simulink model "SmithPredictorEinstellen"  (R2018b)
settings: Solver=VariableStepAuto  StartTime=0.0  StopTime=900*10  FixedStep=0.1  RelTol=1e-3
undefined symbols (not defined in the file or in its folder): s
libraries: cstblocks x12, simulink x6
settings Model: Creator=Adrian Gehrig  LastModifiedBy=Trips
settings SFSimCC: SimUseLocalCustomCode=off
settings RTWCC: RTWUseLocalCustomCode=off
settings CodeAppCC: StateflowObjectComments=on

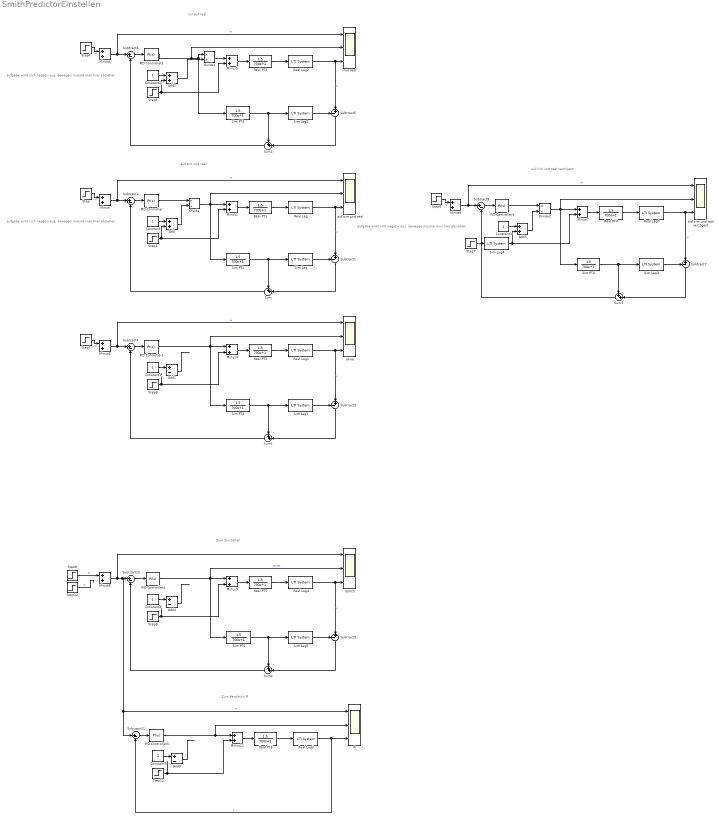
== system SmithPredictorEinstellen ==
  note: Zum Einstellen
  note: nur auf real
  note: aufgabe wirkt sich negativ aus, dewegen müsste man hier abziehen
  note: aufgabe wirkt sich negativ aus, dewegen müsste man hier abziehen
  note: auf sim und real
  note: aufgabe wirkt sich negativ aus, dewegen müsste man hier abziehen
  note: auf sim und real verzögert
  note: Zum Vergleich PI
  Add : Sum
  Add1 : Sum  Inputs=+-
  Add2 : Sum
  Add3 : Sum
  Add4 : Sum  Inputs=+-
  Add5 : Sum  Inputs=+-
  Constant{,1..5} (6 alike) : Constant
  Divide : Product  Inputs=*/
  Divide1 : Product  Inputs=*/
  Divide2 : Product  Inputs=*/
  Minus{,1..9,11} (11 alike) : Sum
  PI : Scope  NumInputPorts=3
  PID Controller{,1..3} (4 alike) : simulink/Continuous/PID Controller  Controller=PI  Form=Ideal  TimeDomain=Continuous-time  SampleTime=-1  IntegratorMethod=Forward Euler  FilterMethod=Forward Euler  ControllerParametersSource=internal  P=1  I=0.00482346678976217  D=0  UseFilter=on  N=100  TunerSelectOption=Transfer Function Based (PID Tuner App)  InitialConditionSource=internal  InitialConditionForIntegrator=0  InitialConditionForFilter=0  DifferentiatorICPrevScaledInput=0  ExternalReset=none  TrackingMode=off  Kt=1  LimitOutput=off  UpperSaturationLimit=inf  LowerSaturationLimit=-inf  LinearizeAsGain=on  AntiWindupMode=none  Kb=1  POutMin=[]  POutMax=[]  IOutMin=[]  IOutMax=[]  DOutMin=[]  DOutMax=[]  NOutMin=[]  NOutMax=[]  SumOutMin=[]  SumOutMax=[]  SaturationOutMin=[]  SaturationOutMax=[]  PParamMin=[]  PParamMax=[]  IParamMin=[]  IParamMax=[]  DParamMin=[]  DParamMax=[]  NParamMin=[]  NParamMax=[]  KbParamMin=[]  KbParamMax=[]  KtParamMin=[]  KtParamMax=[]  KbOutMin=[]  KbOutMax=[]  KtOutMin=[]  KtOutMax=[]  IntegratorOutMin=[]  IntegratorOutMax=[]  FilterOutMin=[]  FilterOutMax=[]  SumI1OutMin=[]  SumI1OutMax=[]  SumI2OutMin=[]  SumI2OutMax=[]  SumI3OutMin=[]  SumI3OutMax=[]  SumI4OutMin=[]  SumI4OutMax=[]  SumDOutMin=[]  SumDOutMax=[]  DifferentiatorOutMin=[]  DifferentiatorOutMax=[]  FilterDiffOutCoefMin=[]  FilterDiffOutCoefMax=[]  ReciprocalOutMin=[]  ReciprocalOutMax=[]  SumDenOutMin=[]  SumDenOutMax=[]  SumNumOutMin=[]  SumNumOutMax=[]  DivideOutMin=[]  DivideOutMax=[]  IntegratorContinuousStateAttributes=''  IntegratorStateMustResolveToSignalObject=off  IntegratorRTWStateStorageClass=Auto  FilterContinuousStateAttributes=''  FilterStateMustResolveToSignalObject=off  FilterRTWStateStorageClass=Auto  ParallelPVariant=Passthrough  IdealPVariant=InternalParameters  IVariant=InternalParameters  DVariant=Disabled  IntegratorVariant=Continuous  SatVariant=Disabled  AWVariant=Passthrough  PCopyVariant=Disabled  TRVariant=Disabled  FdbkBlocksVariant=Forward  IdealPFdbkVariant=Disabled  SatFdbkVariant=Disabled  DerivativeFilterVariant=Disabled  NVariant=Disabled  NCopyVariant=Disabled_SignalSpec  FilterICVariant=Disabled  IntegratorICVariant=InternalICs  ExternalResetVariant=Disabled  TRSumVariant=Passthrough  SumFdbkVariant=Disabled  SumVariant=Sum_PI
  PID Controller4 : simulink/Continuous/PID Controller  Controller=PI  Form=Ideal  TimeDomain=Continuous-time  SampleTime=-1  IntegratorMethod=Forward Euler  FilterMethod=Forward Euler  ControllerParametersSource=internal  P=0.3  I=0.00122023353289823  D=0  UseFilter=on  N=100  TunerSelectOption=Transfer Function Based (PID Tuner App)  InitialConditionSource=internal  InitialConditionForIntegrator=0  InitialConditionForFilter=0  DifferentiatorICPrevScaledInput=0  ExternalReset=none  TrackingMode=off  Kt=1  LimitOutput=off  UpperSaturationLimit=inf  LowerSaturationLimit=-inf  LinearizeAsGain=on  AntiWindupMode=none  Kb=1  POutMin=[]  POutMax=[]  IOutMin=[]  IOutMax=[]  DOutMin=[]  DOutMax=[]  NOutMin=[]  NOutMax=[]  SumOutMin=[]  SumOutMax=[]  SaturationOutMin=[]  SaturationOutMax=[]  PParamMin=[]  PParamMax=[]  IParamMin=[]  IParamMax=[]  DParamMin=[]  DParamMax=[]  NParamMin=[]  NParamMax=[]  KbParamMin=[]  KbParamMax=[]  KtParamMin=[]  KtParamMax=[]  KbOutMin=[]  KbOutMax=[]  KtOutMin=[]  KtOutMax=[]  IntegratorOutMin=[]  IntegratorOutMax=[]  FilterOutMin=[]  FilterOutMax=[]  SumI1OutMin=[]  SumI1OutMax=[]  SumI2OutMin=[]  SumI2OutMax=[]  SumI3OutMin=[]  SumI3OutMax=[]  SumI4OutMin=[]  SumI4OutMax=[]  SumDOutMin=[]  SumDOutMax=[]  DifferentiatorOutMin=[]  DifferentiatorOutMax=[]  FilterDiffOutCoefMin=[]  FilterDiffOutCoefMax=[]  ReciprocalOutMin=[]  ReciprocalOutMax=[]  SumDenOutMin=[]  SumDenOutMax=[]  SumNumOutMin=[]  SumNumOutMax=[]  DivideOutMin=[]  DivideOutMax=[]  IntegratorContinuousStateAttributes=''  IntegratorStateMustResolveToSignalObject=off  IntegratorRTWStateStorageClass=Auto  FilterContinuousStateAttributes=''  FilterStateMustResolveToSignalObject=off  FilterRTWStateStorageClass=Auto  ParallelPVariant=Passthrough  IdealPVariant=InternalParameters  IVariant=InternalParameters  DVariant=Disabled  IntegratorVariant=Continuous  SatVariant=Disabled  AWVariant=Passthrough  PCopyVariant=Disabled  TRVariant=Disabled  FdbkBlocksVariant=Forward  IdealPFdbkVariant=Disabled  SatFdbkVariant=Disabled  DerivativeFilterVariant=Disabled  NVariant=Disabled  NCopyVariant=Disabled_SignalSpec  FilterICVariant=Disabled  IntegratorICVariant=InternalICs  ExternalResetVariant=Disabled  TRSumVariant=Passthrough  SumFdbkVariant=Disabled  SumVariant=Sum_PI
  PID Controller5 : simulink/Continuous/PID Controller  Controller=PI  Form=Ideal  TimeDomain=Continuous-time  SampleTime=-1  IntegratorMethod=Forward Euler  FilterMethod=Forward Euler  ControllerParametersSource=internal  P=0.3  I=0.00122496125356266  D=0  UseFilter=on  N=100  TunerSelectOption=Transfer Function Based (PID Tuner App)  InitialConditionSource=internal  InitialConditionForIntegrator=0  InitialConditionForFilter=0  DifferentiatorICPrevScaledInput=0  ExternalReset=none  TrackingMode=off  Kt=1  LimitOutput=off  UpperSaturationLimit=inf  LowerSaturationLimit=-inf  LinearizeAsGain=on  AntiWindupMode=none  Kb=1  POutMin=[]  POutMax=[]  IOutMin=[]  IOutMax=[]  DOutMin=[]  DOutMax=[]  NOutMin=[]  NOutMax=[]  SumOutMin=[]  SumOutMax=[]  SaturationOutMin=[]  SaturationOutMax=[]  PParamMin=[]  PParamMax=[]  IParamMin=[]  IParamMax=[]  DParamMin=[]  DParamMax=[]  NParamMin=[]  NParamMax=[]  KbParamMin=[]  KbParamMax=[]  KtParamMin=[]  KtParamMax=[]  KbOutMin=[]  KbOutMax=[]  KtOutMin=[]  KtOutMax=[]  IntegratorOutMin=[]  IntegratorOutMax=[]  FilterOutMin=[]  FilterOutMax=[]  SumI1OutMin=[]  SumI1OutMax=[]  SumI2OutMin=[]  SumI2OutMax=[]  SumI3OutMin=[]  SumI3OutMax=[]  SumI4OutMin=[]  SumI4OutMax=[]  SumDOutMin=[]  SumDOutMax=[]  DifferentiatorOutMin=[]  DifferentiatorOutMax=[]  FilterDiffOutCoefMin=[]  FilterDiffOutCoefMax=[]  ReciprocalOutMin=[]  ReciprocalOutMax=[]  SumDenOutMin=[]  SumDenOutMax=[]  SumNumOutMin=[]  SumNumOutMax=[]  DivideOutMin=[]  DivideOutMax=[]  IntegratorContinuousStateAttributes=''  IntegratorStateMustResolveToSignalObject=off  IntegratorRTWStateStorageClass=Auto  FilterContinuousStateAttributes=''  FilterStateMustResolveToSignalObject=off  FilterRTWStateStorageClass=Auto  ParallelPVariant=Passthrough  IdealPVariant=InternalParameters  IVariant=InternalParameters  DVariant=Disabled  IntegratorVariant=Continuous  SatVariant=Disabled  AWVariant=Passthrough  PCopyVariant=Disabled  TRVariant=Disabled  FdbkBlocksVariant=Forward  IdealPFdbkVariant=Disabled  SatFdbkVariant=Disabled  DerivativeFilterVariant=Disabled  NVariant=Disabled  NCopyVariant=Disabled_SignalSpec  FilterICVariant=Disabled  IntegratorICVariant=InternalICs  ExternalResetVariant=Disabled  TRSumVariant=Passthrough  SumFdbkVariant=Disabled  SumVariant=Sum_PI
  Real Lag{,1..5} (6 alike) : cstblocks/LTI System  sys=exp(-420*s)  IC=[]
  Real PT{1..6} (6 alike) : TransferFcn  Numerator=[1.5]  Denominator=[700 1]
  Sim Lag{,1..4} (5 alike) : cstblocks/LTI System  sys=exp(-400*s)  IC=[]
  Sim Lag5 : cstblocks/LTI System  sys=exp(-420*s)  IC=[]
  Sim PT{1..5} (5 alike) : TransferFcn  Numerator=[1.5]  Denominator=[700 1]
  Smith : Scope  NumInputPorts=3
  Step{,2,4,6,8} (5 alike) : Step  SampleTime=0
  Step{1,3,5,7,9,11} (6 alike) : Step  Time=5000  SampleTime=0
  Step12 : Step  Time=3000  SampleTime=0
  Subtract{1,3,5,7,9} (5 alike) : Sum  Inputs=-+|
  Subtract{2,4,6,8,10..11} (6 alike) : Sum  Inputs=|+-
  Sum{,1..4} (5 alike) : Sum  Inputs=++|
  "auf sim und real " : Scope  NumInputPorts=3
  auf sim und real verzögert : Scope  NumInputPorts=3
  nur real : Scope  NumInputPorts=3
  ohne : Scope  NumInputPorts=3
  wires:
  Sim PT1/1 -> Sum/1, Sim Lag/1
  Subtract1/1 -> Sum/2
  Sim Lag/1 -> Subtract1/1
  Sum/1 -> Subtract2/2
  Divide/1 -> "auf sim und real "/2, Minus1/1, Sim PT1/1
  Minus/1 -> "auf sim und real "/1, Subtract2/1  "w"
  Subtract2/1 -> PID Controller/1
  Real Lag/1 -> "auf sim und real "/3, Subtract1/2  "y"
  Step/1 -> Minus/1  "w"
  Step1/1 -> Add/2, Minus1/2
  Real PT1/1 -> Real Lag/1
  Minus1/1 -> Real PT1/1
  PID Controller/1 -> Divide/1
  Add/1 -> Divide/2
  Constant/1 -> Add/1
  Step3/1 -> Minus3/2
  Sim PT2/1 -> Sum1/1, Sim Lag1/1
  Real PT2/1 -> Real Lag1/1
  PID Controller1/1 -> Sim PT2/1, ohne/2, Minus3/1
  Real Lag1/1 -> ohne/3, Subtract3/2  "y"
  Minus2/1 -> ohne/1, Subtract4/1  "w"
  Step2/1 -> Minus2/1  "w"
  Minus3/1 -> Real PT2/1
  Sim Lag1/1 -> Subtract3/1
  Sum1/1 -> Subtract4/2
  Subtract3/1 -> Sum1/2
  Constant1/1 -> Add1/1
  Subtract4/1 -> PID Controller1/1
  Add1/1 -> ?
  Step5/1 -> Add2/2, Minus5/2
  Sim PT3/1 -> Sum2/1, Sim Lag2/1
  Real PT3/1 -> Real Lag2/1
  Real Lag2/1 -> nur real/3, Subtract5/2  "y"
  Minus4/1 -> nur real/1, Subtract6/1  "w"
  Step4/1 -> Minus4/1  "w"
  Minus5/1 -> Real PT3/1
  Sim Lag2/1 -> Subtract5/1
  Sum2/1 -> Subtract6/2
  Subtract5/1 -> Sum2/2
  PID Controller2/1 -> Sim PT3/1, Divide1/1, nur real/2
  Constant2/1 -> Add2/1
  Subtract6/1 -> PID Controller2/1
  Divide1/1 -> Minus5/1
  Add2/1 -> Divide1/2
  Step7/1 -> Sim Lag4/1
  Sim PT4/1 -> Sum3/1, Sim Lag3/1
  Real PT4/1 -> Real Lag3/1
  Real Lag3/1 -> auf sim und real verzögert/3, Subtract7/2  "y"
  Minus6/1 -> auf sim und real verzögert/1, Subtract8/1  "w"
  Step6/1 -> Minus6/1  "w"
  Minus7/1 -> Real PT4/1
  Sim Lag3/1 -> Subtract7/1
  Sum3/1 -> Subtract8/2
  Subtract7/1 -> Sum3/2
  Divide2/1 -> auf sim und real verzögert/2, Minus7/1, Sim PT4/1
  Add3/1 -> Divide2/2
  PID Controller3/1 -> Divide2/1
  Constant3/1 -> Add3/1
  Subtract8/1 -> PID Controller3/1
  Sim Lag4/1 -> Add3/2, Minus7/2
  PID Controller4/1 -> Sim PT5/1, Smith/2, Minus9/1  "smith"
  Constant4/1 -> Add4/1
  Add4/1 -> ?
  Sum4/1 -> Subtract10/2
  Subtract9/1 -> Sum4/2
  Sim Lag5/1 -> Subtract9/1
  Minus9/1 -> Real PT5/1
  Real Lag4/1 -> Smith/3, Subtract9/2  "y"
  Step8/1 -> Minus8/1  "w"
  Real PT5/1 -> Real Lag4/1
  Sim PT5/1 -> Sum4/1, Sim Lag5/1
  Subtract10/1 -> PID Controller4/1
  Step9/1 -> Minus9/2
  Real PT6/1 -> Real Lag5/1
  Step11/1 -> Minus11/2
  Subtract11/1 -> PID Controller5/1
  Minus11/1 -> Real PT6/1
  Minus8/1 -> Subtract11/1, PI/1, Subtract10/1, Smith/1  "w"
  Real Lag5/1 -> Subtract11/2, PI/3  "y"
  Add5/1 -> ?
  Constant5/1 -> Add5/1
  PID Controller5/1 -> PI/2, Minus11/1
  Step12/1 -> ?  "w"
